simulink model "alinea6"  (R2017b)
settings: Solver=VariableStepAuto  StartTime=0.0  StopTime=10.0  RelTol=1e-3
settings Model: Creator=Rita Monteiro  LastModifiedBy=Rita Monteiro

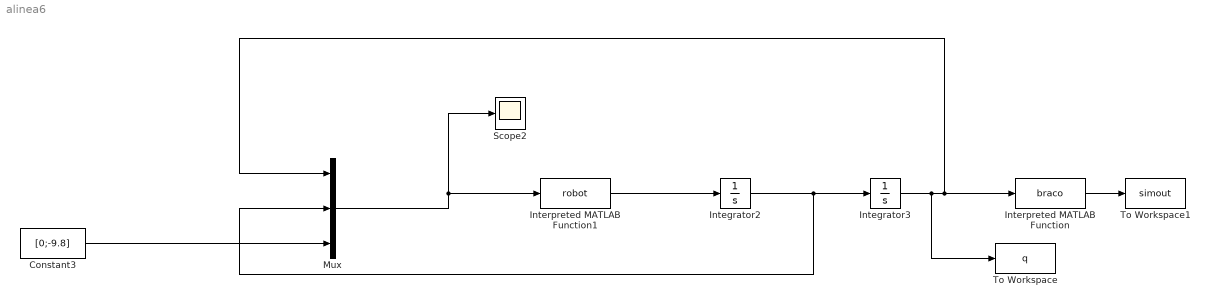
== system alinea6 ==
  Constant3 : Constant  Value=[0;-9.8]  VectorParams1D=off
  Integrator2 : Integrator  InitialCondition=[0;0]
  Integrator3 : Integrator  InitialCondition=[pi/2;pi/4]
  Interpreted MATLAB Function : MATLABFcn  MATLABFcn=braco  OutputDimensions=1
  Interpreted MATLAB Function1 : MATLABFcn  MATLABFcn=robot  OutputDimensions=2
  Mux : Mux  Inputs=3
  Scope2 : Scope
  To Workspace : ToWorkspace  VariableName=q
  To Workspace1 : ToWorkspace  VariableName=simout  SaveFormat=Timeseries  SampleTime=-1
  wires:
  Mux/1 -> Scope2/1, Interpreted MATLAB Function1/1
  Integrator2/1 -> Mux/2, Integrator3/1
  Constant3/1 -> Mux/3
  Interpreted MATLAB Function1/1 -> Integrator2/1
  Integrator3/1 -> Interpreted MATLAB Function/1, Mux/1, To Workspace/1
  Interpreted MATLAB Function/1 -> To Workspace1/1
